simulink model "EnablePort1"  (R2017b)
settings: Solver=FixedStepDiscrete  StartTime=0.0  StopTime=10.0  FixedStep=0.200000  RelTol=1e-3
model workspace (MAT data in the model file):
  input_struct.time = [0; 0.2; 0.4; 0.6; 0.8; 1; 1.2; 1.4; 1.6; 1.8; 2; 2.2; 2.4; 2.6; 2.8; 3; 3.2; 3.4; 3.6; 3.8; 4; 4.2; 4.4; 4.6; 4.8; 5; 5.2; 5.4; 5.6; 5.8; 6; 6.2; 6.4; 6.6; 6.8; 7; 7.2; 7.4; 7.6; 7.8; 8; 8.2; 8.4; 8.6; 8.8; 9; 9.2; 9.4; 9.6; 9.8; 10; 10.2; 10.4; 10.6; 10.8; 11; 11.2; 11.4; 11.6; 11.8; 12; 12.2; 12.4; 12.6; 12.8; 13; 13.2; 13.4; 13.6; 13.8; 14; 14.2; 14.4; 14.6; 14.8; 15; 15.2; 15.4; 15.6; 15.8; 16; 16.2; 16.4; 16.6; 16.8; 17; 17.2; 17.4; 17.6; 17.8; 18; 18.2; 18.4; 18.6; 18.8; 19; 19.2; 19.4; 19.6; 19.8]
  input_struct.signals(1).name = 'In1'
  input_struct.signals(1).values = [36.49153289; -28.3750938036; 97.3853539924; -83.2027408488; -49.9388227277; 62.269323063; -83.1153792244; 6.25079274837; 60.1245958296; 47.7646483842; -71.6674039395; -12.421148419; -29.9239255173; -4.30050056046; 17.4806800248; -70.8388609561; 81.0661214489; 28.0388496664; -67.4120857119; 13.1821182003; 86.3232273954; 56.6203767369; 37.1374273958; -6.75614300345; -47.9363808667; 13.8536342154; -50.2458674224; -36.1396816958; 82.1604464434; 77.0440081989; 58.9178848332; 85.1619614334; -64.2320098448; 3.50822964729; 25.4010632819; 82.6364691802; 32.7936507678; -22.1614354015; 48.0015162832; 63.5269719417; 20.0689586353; -83.0005870995; 84.471600218; -89.2804369367; 5.40499053547; -76.2293446761; -23.9714019518; 62.566506603; -51.1808168857; 76.8845318187; 42.5293589518; -24.3703123836; -50.2160778008; -49.4292509521; 53.4487189054; -90.0276229906; 37.0577135218; 24.0556244302; 49.3369259937; 95.4511296691; -23.2172974679; -47.9588795373; 75.4939072028; 61.2191967021; -7.77578404406; -81.8076624152; 12.8537650546; -62.5234221703; 6.33791717895; -28.9933356453; -37.0432990489; 45.3482937685; 3.15457162671; 58.1289795825; -59.1014837282; 35.621215512; -89.5028914724; 60.2344724725; 35.7137277639; 89.2017890168; -81.688371425; 81.6876741156; 1.99060741064; 22.980713028; -36.7857598228; -84.5025036969; 70.1228132007; -71.0946186103; -25.9028414692; 24.4782866163; 99.5103804863; 3.46882664914; 98.1022430301; -54.6931074888; -20.398962716; 39.3137379023; -87.0718481093; 49.5323164757; -15.9199137534; 62.2634840476]
  input_struct.signals(1).dimensions = 1
  input_struct.signals(2).name = 'Enable'
  input_struct.signals(2).values = [-24.0789428459; -36.1864359566; 97.2102133453; 43.6361810419; -17.363328286; -80.2739525514; 46.9118250333; 27.4612580707; -85.2316246528; -75.8983667196; 96.3192417833; -0.64011564417; -95.517269112; -89.2336902061; -71.8252404796; 78.694862348; -6.83598537679; 12.1713476267; -1.10873052332; -86.4429023028; 79.5293084747; -42.2869382237; -46.1906370493; 18.8388350861; -4.82419518874; -26.3377923853; 31.1222180993; 87.6400811609; 24.0850371568; -43.4319816771; -58.9637496134; -12.1731836812; -94.5499560678; 75.2368671921; 22.0184492549; -59.2815239425; 3.98336495808; -89.23513957; 72.4374862234; -11.4130667892; 9.60183146713; 13.3721663578; 36.0789982429; -25.7242843814; -84.3542581629; -8.72985526999; -90.4312399679; 47.6513984054; -92.3996929208; 90.8488648719; 48.4744668927; 87.4899134081; 2.67279723153; -51.8190401845; -48.0069442566; 51.7948322684; 98.6685527683; -28.6588500151; 50.5715682206; -77.9903005775; 19.4090459229; -13.8809599359; 46.1436034643; -47.7647658857; -81.0384636833; -9.80730214177; 28.0149020535; -73.5922365262; -9.43551403519; 30.4399197896; 65.3996663116; -38.384618316; -19.527284199; 76.8462632093; 40.115902011; -51.6255409705; 51.9663631439; -41.8148525613; -44.5122562089; -98.7784393947; -25.0577717709; -12.6134438536; -39.1403062317; -41.8279338782; -51.496738223; 87.3367220045; 72.0380481654; -20.5543479124; -4.11617912828; 12.999218619; -2.07612209069; -46.0376734652; 97.9480284124; -63.2648607468; 72.3313449848; -93.4734855787; -33.6083960827; 49.7493991566; 28.8732916363; -66.1524074697]
  input_struct.signals(2).dimensions = 1
settings Model: Creator=hbourbou  LastModifiedBy=hbourbou
settings DataIOCC: SaveFormat=StructureWithTime
settings OptimizationCC: LifeSpan=inf
settings DebuggingCC: SFExecutionAtInitializationDiag=none
settings HardwareCC: ProdBitPerSizeT=32  ProdBitPerPtrDiffT=32  ProdWordSize=32  ProdHWDeviceType=Specified
settings CodeAppCC: StateflowObjectComments=on

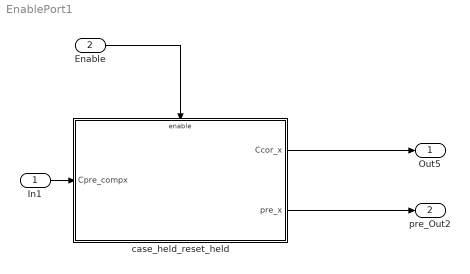
== system EnablePort1 ==
  In1 : Inport
  Enable : Inport  Port=2
  case_held_reset_held : Subsystem  TreatAsAtomicUnit=on
  Out5 : Outport
  pre_Out2 : Outport  Port=2
  wires:
  In1/1 -> case_held_reset_held/1(Cpre_compx)
  case_held_reset_held/1(Ccor_x) -> Out5/1
  case_held_reset_held/2(pre_x) -> pre_Out2/1
  Enable/1 -> case_held_reset_held/Enable

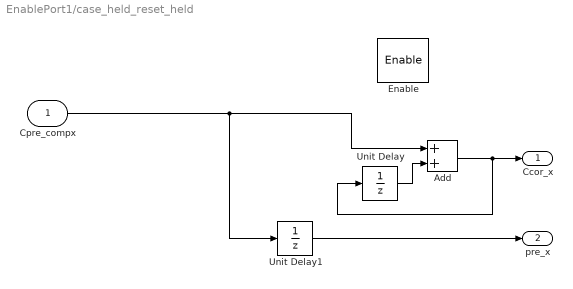
== system EnablePort1/case_held_reset_held ==
  Cpre_compx : Inport  OutDataTypeStr=double  PortDimensions=[1]
  Enable : EnablePort
  Add : Sum
  Unit Delay : UnitDelay  SampleTime=-1.0000000000000000
  Unit Delay1 : UnitDelay  SampleTime=-1
  Ccor_x : Outport  OutputWhenDisabled=reset  InitialOutput=0
  pre_x : Outport  Port=2  InitialOutput=0
  wires:
  Cpre_compx/1 -> Unit Delay1/1, Add/1
  Add/1 -> Unit Delay/1, Ccor_x/1
  Unit Delay/1 -> Add/2
  Unit Delay1/1 -> pre_x/1
